simulink model "VENTO_AUREO"  (R2024a)
settings: Solver=VariableStepAuto  StartTime=0.0  StopTime=3600  RelTol=1e-3
settings Model: Creator=emanuele  LastModifiedBy=emanuele

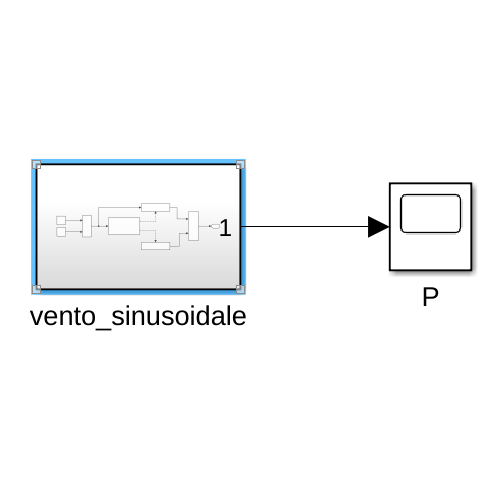
[thumbnail: Simulink's stored preview of the top-level diagram]
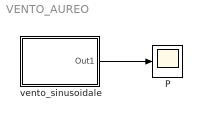
== system VENTO_AUREO ==
  P : Scope
  vento_sinusoidale : Subsystem
  wires:
  vento_sinusoidale/1(Out1) -> P/1

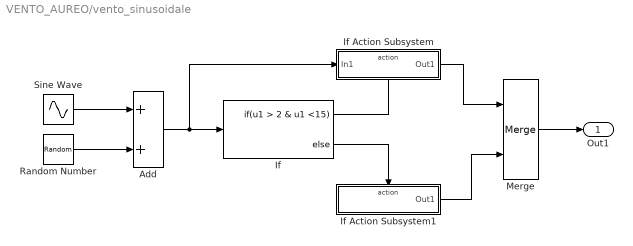
== system VENTO_AUREO/vento_sinusoidale ==
  Add : Sum
  If : If  IfExpression=u1 > 2 & u1 <15
  If Action Subsystem : Subsystem  TreatAsAtomicUnit=on
  If Action Subsystem1 : Subsystem  TreatAsAtomicUnit=on
  Merge : Merge
  Random Number : RandomNumber  Variance=2  SampleTime=1
  Sine Wave : Sin  Amplitude=5.5  Bias=8.5  Frequency=2*pi/90  SampleTime=0
  Out1 : Outport
  wires:
  If/2 -> If Action Subsystem1/Action
  Add/1 -> If Action Subsystem/1(In1), If/1
  Sine Wave/1 -> Add/1
  Merge/1 -> Out1/1
  Random Number/1 -> Add/2
  If Action Subsystem/1(Out1) -> Merge/1
  If Action Subsystem1/1(Out1) -> Merge/2
  If/1 -> If Action Subsystem/Action

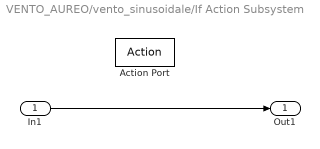
== system VENTO_AUREO/vento_sinusoidale/If Action Subsystem ==
  In1 : Inport
  Action Port : ActionPort  ActionPortLabel=if(u1 > 2 & u1 <15)
  Out1 : Outport
  wires:
  In1/1 -> Out1/1

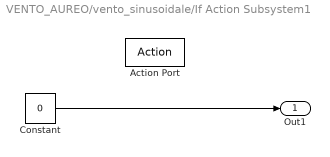
== system VENTO_AUREO/vento_sinusoidale/If Action Subsystem1 ==
  Action Port : ActionPort  ActionPortLabel=else
  Constant : Constant  Value=0
  Out1 : Outport
  wires:
  Constant/1 -> Out1/1
